simulink model "TestDelay"  (R2014b)
settings: Solver=ode3  SolverMode=SingleTasking  StartTime=0.0  StopTime=0.1  FixedStep=fpgaclk  RelTol=1e-3
undefined symbols (not defined in the file or in its folder): fpgaclk
libraries: xbsIndex_r4 x7, simulink x1, MyFunctions x1
settings Model: Creator=gnaylor  LastModifiedBy=gnaylor

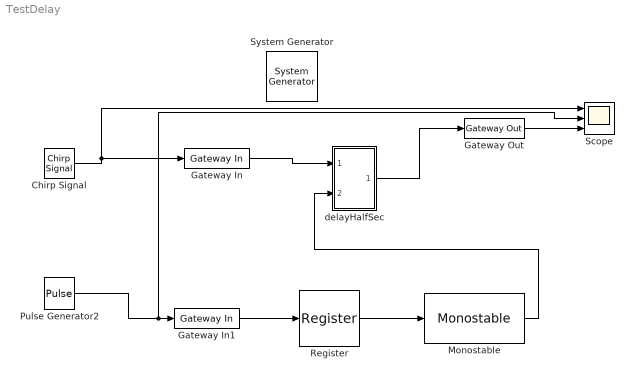
== system TestDelay ==
  " System Generator" : xbsIndex_r4/ System Generator  Tag=genX  xilinxfamily=zynq  part=xc7z010  speed=-1  package=clg225  synthesis_tool=XST  clock_wrapper=Clock Enables  directory=../SysgenOutput/TE0722/ToneDetect2  proj_type=Project Navigator  Synth_file=XST Defaults  Impl_file=ISE Defaults  testbench=off  simulink_period=fpgaclk  sysclk_period=1e9*fpgaclk  dcm_input_clock_period=100  incr_netlist=off  trim_vbits=Everywhere in SubSystem  dbl_ovrd=According to Block Masks  core_generation=According to Block Masks  run_coregen=off  deprecated_control=off  eval_field=0  block_type=sysgen
      settings: block_version=8.2.02
  Chirp Signal : simulink/Sources/Chirp Signal  f1=1e3  T=0.1  f2=1e4
  Gateway In : xbsIndex_r4/Gateway In  gui_display_data_type=Fixed-point  arith_type="Signed  (2's comp)"  n_bits=16  bin_pt=14  preci_type=Single  exp_width=8  frac_width=24  rows=1  columns=1  quantization="Round  (unbiased: +/- Inf)"  overflow=Saturate  period=fpgaclk  UseAsADC=off  ADCChannel='1'  interface=None  automatic_assignment=on  address_offset=hex2dec('00')  intf_name=''  intf_description=''  default_value=0  timing_constraint=None  locs_specified=off  LOCs={}  io_standard={}  inherit_from_input=off  hdl_port=on  dbl_ovrd=off  block_type=gatewayin
  Gateway In1 : xbsIndex_r4/Gateway In  gui_display_data_type=Boolean  arith_type=Boolean  n_bits=16  bin_pt=14  preci_type=Single  exp_width=8  frac_width=24  rows=1  columns=1  quantization="Round  (unbiased: +/- Inf)"  overflow=Saturate  period=fpgaclk  UseAsADC=off  ADCChannel='1'  interface=None  automatic_assignment=on  address_offset=hex2dec('00')  intf_name=''  intf_description=''  default_value=0  timing_constraint=None  locs_specified=off  LOCs={}  io_standard={}  inherit_from_input=off  hdl_port=on  dbl_ovrd=off  block_type=gatewayin
  Gateway Out : xbsIndex_r4/Gateway Out  inherit_from_input=off  hdl_port=on  rows=1  columns=1  UseAsDAC=off  DACChannel='1'  interface=None  automatic_assignment=on  address_offset=hex2dec('00')  intf_name=''  intf_description=''  timing_constraint=None  locs_specified=off  LOCs={}  io_standard={}  block_type=gatewayout
  Monostable : MyFunctions/Monostable
  Pulse Generator2 : DiscretePulseGenerator  PulseType=Time based  Period=100*fpgaclk  PulseWidth=10
  Register : xbsIndex_r4/Register  init=0  rst=off  en=off  dbl_ovrd=off  block_type=register
  Scope : Scope  NumInputPorts=3
      settings: YMin=-5~-5~-5  YMax=5~5~5
  delayHalfSec : Subsystem
  wires:
  Chirp Signal/1 -> Scope/1, Gateway In/1
  Gateway Out/1 -> Scope/3
  Pulse Generator2/1 -> Scope/2, Gateway In1/1
  Gateway In/1 -> delayHalfSec/1(In1)
  Gateway In1/1 -> Register/1
  Monostable/1 -> delayHalfSec/2(Strobe)
  delayHalfSec/1(Out1) -> Gateway Out/1
  Register/1 -> Monostable/1

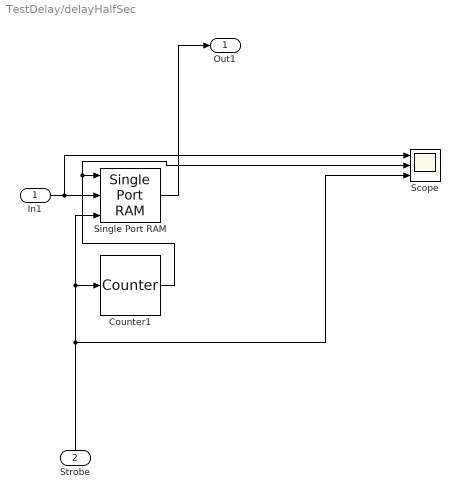
== system TestDelay/delayHalfSec ==
  In1 : Inport
  Strobe : Inport  Port=2
  Counter1 : xbsIndex_r4/Counter  cnt_type=Free Running  cnt_to=Inf  operation=Up  start_count=0  cnt_by_val=1  arith_type=Unsigned  n_bits=12  bin_pt=0  load_pin=off  rst=off  en=on  explicit_period=on  period=fpgaclk  use_behavioral_HDL=off  implementation=Fabric  dbl_ovrd=off  block_type=counter
  Scope : Scope  NumInputPorts=3
      settings: YMin=0~0~0  YMax=0.6~6000~1
  Single Port RAM : xbsIndex_r4/Single Port RAM  depth=4096  initVector=zeros(4096,1)  distributed_mem=Block RAM  write_mode=Read Before Write  rst=off  init_reg=0  en=off  latency=1  optimize=Area  dbl_ovrd=off  block_type=spram
  Out1 : Outport
  wires:
  Single Port RAM/1 -> Out1/1
  Strobe/1 -> Single Port RAM/3, Counter1/1, Scope/3
  Counter1/1 -> Scope/2, Single Port RAM/1
  In1/1 -> Scope/1, Single Port RAM/2
